simulink model "my_loop_model"  (R2025b)
settings: Solver=VariableStepAuto  StartTime=0.0  StopTime=10.0  RelTol=1e-3
settings Model: Creator=lab  LastModifiedBy=lab

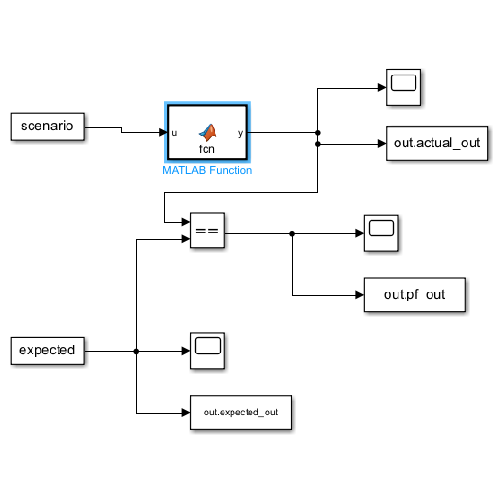
[thumbnail: Simulink's stored preview of the top-level diagram]
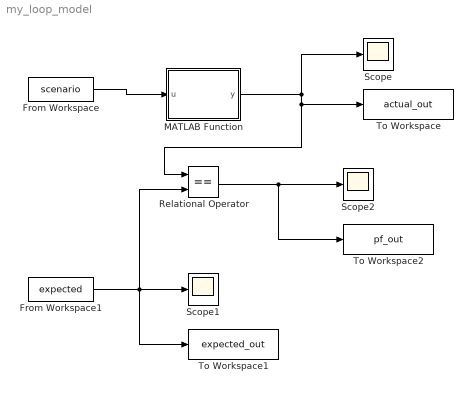
== system my_loop_model ==
  From Workspace : FromWorkspace  VariableName=scenario  Interpolate=off  OutputAfterFinalValue=Holding final value
  From Workspace1 : FromWorkspace  VariableName=expected  Interpolate=off  OutputAfterFinalValue=Holding final value
  MATLAB Function : MATLAB Function  TreatAsAtomicUnit=on
  Relational Operator : RelationalOperator  Operator===  OutDataTypeStr=boolean  RndMeth=Simplest  InputSameDT=off
  Scope : Scope
  Scope1 : Scope
  Scope2 : Scope
      settings: DataLoggingVariableName=ScopeData2
  To Workspace : ToWorkspace  VariableName=actual_out  SaveFormat=Timeseries  SampleTime=-1
  To Workspace1 : ToWorkspace  VariableName=expected_out  SaveFormat=Timeseries  SampleTime=-1
  To Workspace2 : ToWorkspace  VariableName=pf_out  SaveFormat=Timeseries  SampleTime=-1
  wires:
  From Workspace/1 -> MATLAB Function/1(u)
  MATLAB Function/1(y) -> Relational Operator/1, To Workspace/1, Scope/1
  From Workspace1/1 -> Relational Operator/2, Scope1/1, To Workspace1/1
  Relational Operator/1 -> To Workspace2/1, Scope2/1

== matlab function my_loop_model/MATLAB Function ==
  data: u input; y output
function y = fcn(u)
coder.extrinsic('llm_step');

y = 0;
tmp = llm_step(double(u));

if isempty(tmp)
    y = 0;
else
    y = double(tmp);
end
end
